simulink model "withcontrolertwoarea"  (R2024a)
settings: Solver=FixedStepAuto  StartTime=0.0  StopTime=20  FixedStep=0.01  RelTol=1e-3
settings Model: Creator=farza  LastModifiedBy=farza

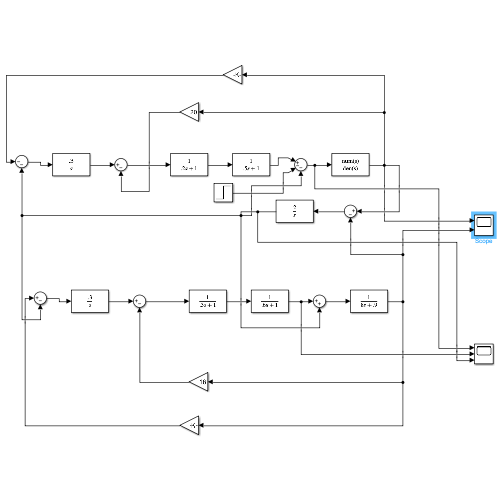
[thumbnail: Simulink's stored preview of the top-level diagram]
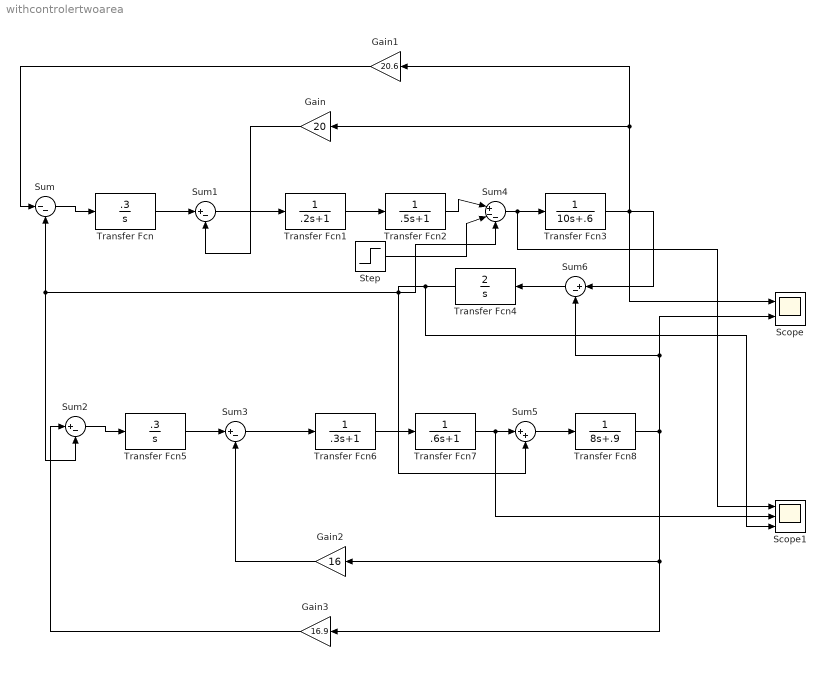
== system withcontrolertwoarea ==
  Gain : Gain  Gain=20
  Gain1 : Gain  Gain=20.6
  Gain2 : Gain  Gain=16
  Gain3 : Gain  Gain=16.9
  Scope : Scope  NumInputPorts=2
  Scope1 : Scope  NumInputPorts=3
  Step : Step  Before=.1875  After=.1875  SampleTime=0
  Sum : Sum  Inputs=|--
  Sum{1..3,6} (4 alike) : Sum  Inputs=|+-
  Sum4 : Sum  Inputs=|+--
  Sum5 : Sum  Inputs=|++
  Transfer Fcn : TransferFcn  Numerator=[.3]  Denominator=[1 0]
  Transfer Fcn1 : TransferFcn  Denominator=[.2 1]
  Transfer Fcn2 : TransferFcn  Denominator=[.5 1]
  Transfer Fcn3 : TransferFcn  Denominator=[10 .6]
  Transfer Fcn4 : TransferFcn  Numerator=[2]  Denominator=[1 0]
  Transfer Fcn5 : TransferFcn  Numerator=[.3]  Denominator=[1 0]
  Transfer Fcn6 : TransferFcn  Denominator=[.3 1]
  Transfer Fcn7 : TransferFcn  Denominator=[.6 1]
  Transfer Fcn8 : TransferFcn  Denominator=[8 .9]
  wires:
  Sum4/1 -> Scope1/1, Transfer Fcn3/1
  Sum/1 -> Transfer Fcn/1
  Transfer Fcn/1 -> Sum1/1
  Transfer Fcn1/1 -> Transfer Fcn2/1
  Transfer Fcn2/1 -> Sum4/1
  Sum1/1 -> Transfer Fcn1/1
  Transfer Fcn3/1 -> Gain1/1, Gain/1, Scope/1, Sum6/1
  Gain/1 -> Sum1/2
  Gain1/1 -> Sum/1
  Sum6/1 -> Transfer Fcn4/1
  Transfer Fcn8/1 -> Scope/2, Sum6/2, Gain3/1, Gain2/1
  Transfer Fcn7/1 -> Scope1/2, Sum5/1
  Sum3/1 -> Transfer Fcn6/1
  Gain2/1 -> Sum3/2
  Transfer Fcn6/1 -> Transfer Fcn7/1
  Sum2/1 -> Transfer Fcn5/1
  Gain3/1 -> Sum2/1
  Sum5/1 -> Transfer Fcn8/1
  Transfer Fcn5/1 -> Sum3/1
  Transfer Fcn4/1 -> Scope1/3, Sum4/3, Sum5/2, Sum/2, Sum2/2
  Step/1 -> Sum4/2
